simulink model "SF049A_LoaMgr"  (R2013b)
settings: Solver=FixedStepDiscrete  SolverMode=SingleTasking  StartTime=0.0  StopTime=1  FixedStep=0.002  RelTol=1e-3
undefined symbols (not defined in the file): CURRMEASLOAMTGTNMASK_CNT_U08, IVTRLOAMTGTNMASK_CNT_U08, LoaCtrldShtdwn, LoaCurrMeasIdptSigNrFlt, LoaHwTqIdptSigNrFlt, LoaImdtShtdwn, LoaIvtrIdptSigNrFlt, LOAMAXSLEW_ULSPERSEC_F32, LoaMgrCurrIvtrMtgtnRate, LoaMgrCurrIvtrMtgtnSca, LoaMgrCurrIvtrMtgtnScaZeroEna, LoaMgrCurrMeasIdptSig0Resp, LoaMgrCurrMeasIdptSig1Resp, LoaMgrCurrMeasIdptSig2Resp, LoaMgrCurrMeasIdptSigFltThd, LoaMgrCurrMeasMtgtnRate, LoaMgrCurrMeasMtgtnSca, LoaMgrCurrMeasMtgtnScaZeroEna, LoaMgrFadeOutStRate, LoaMgrHwTqIdptSig0NoTqLoaResp, LoaMgrHwTqIdptSig1NoTqLoaResp, LoaMgrHwTqIdptSig2Resp, LoaMgrHwTqIdptSig4Resp, LoaMgrHwTqIdptSigFltThd, LoaMgrHwTqLoaAvlResp, LoaMgrIvtrIdptSig0Resp, LoaMgrIvtrIdptSig1Resp, LoaMgrIvtrIdptSig2Resp, LoaMgrIvtrIdptSigFltThd, LoaMgrIvtrMtgtnRate, LoaMgrIvtrMtgtnSca, LoaMgrIvtrMtgtnScaZeroEna, LoaMgrLimdStRate, LoaMgrLimdStSca, LoaMgrMotAgAvlSnsrlsResp, LoaMgrMotAgIdptSig0NoSnsrlsResp, LoaMgrMotAgIdptSig1NoSnsrlsResp, LoaMgrMotAgIdptSig2Resp, LoaMgrMotAgIdptSig3Resp, LoaMgrMotAgIdptSigFltThd, LoaMgrMotAgMtgtnRate, LoaMgrMotAgMtgtnSca, LoaMgrMotAgMtgtnScaZeroEna, LoaMotAgIdptSigNrFlt, LOASCAONE_ULS_F32, LOASCAZERO_ULS_F32, LoaSt1, LOASTIMDTSHTDWN_CNT_U08, LOASTNORM_CNT_U08, LOASTSWMTGTN_CNT_U08, MAXCURRMEASIDPTSIGALLWD_CNT_U08, MAXHWTQIDPTSIGALLWD_CNT_U08, MAXIVTRIDPTSIGALLWD_CNT_U08, MAXMOTAGMECLIDPTSIGALLWD_CNT_U08, NODEBSTEP_CNT_U16, NtcSts1, SigQlfr1
libraries: simulink x30, NxtrMin x4, NxtrMax x4, NxtrLim x2
(part 5 of 7)

== system SF049A_LoaMgr/LoaMgr/LoaMgrPer1/Request_Responses/InvtrResp ==
  note: SWITCH IvtrIdptMin
      |     CASE 2
      |         CurrMeasResp = LoaMgrIvtrIdptSig2Resp
      |     CASE 1
      |          CurrMeasResp = LoaMgrIvtrIdptSig1Resp
      |     CASE ELSE
      |          CurrMeasResp = LoaMgrIvtrIdptSig0Resp
      | ENDSWITCH
  IvtrIdptMin : Inport  RequirementInfo={} %GIDa_2f7698e0_eca9_423b_adb0_11e1919669ef
  Constant : Constant  RequirementInfo="{'linktype_rmi_doors' '00012fd5 (/E-STEER Core/SubSystem Specifications/Application Functions - EA4/SF049A Loss of Assist Manager)' '#SF049A_128' 'true' 'REQ:  SF049A_128' '' } %GIDa_c2727e40_acbb_4c51_8514_00a2f788091d"  Value=LoaMgrIvtrIdptSig2Resp
  Constant1 : Constant  RequirementInfo="{'linktype_rmi_doors' '00012fd5 (/E-STEER Core/SubSystem Specifications/Application Functions - EA4/SF049A Loss of Assist Manager)' '#SF049A_128' 'true' 'REQ:  SF049A_128' '' } %GIDa_9020f9ee_b1a9_4c7e_bd34_28530cfb2ca8"  Value=LoaMgrIvtrIdptSig1Resp
  Constant2 : Constant  RequirementInfo="{'linktype_rmi_doors' '00012fd5 (/E-STEER Core/SubSystem Specifications/Application Functions - EA4/SF049A Loss of Assist Manager)' '#SF049A_128' 'true' 'REQ:  SF049A_128' '' } %GIDa_e0ea4ff4_d281_47bc_ab32_13335c3cc295"  Value=LoaMgrIvtrIdptSig0Resp
  CopyRight2 : Subsystem  Description=|  mask(Copyright Information){none=on}
      | Copyright info block.                                               
      |                                                                     
      | Place copyright information at the top of every subsystem in design.
      mask prompts: none "No parameters"
      mask help: Place copyright information at the top of every subsystem in design.
      mask Display:
      | NxtrConf = 'Nexteer Confidential';
      | 
      | sys = bdroot; %handle for the current model ("system")
      | first = get_param(sys,'Created');
      | first = first(end-3:end);  %year is last four digits
      | 
      | last = get_param(sys,'LastModifiedDate');
      | if isempty(last)
      |     last = datestr(now,'yyyy');
      | else
      |     last = last(end-3:end);
      | end
      | 
      | if strcmp(first,last)
      |     fprintf('%s -- Copyright %s Nexteer',NxtrConf,first)
      | else
      |     fprintf('%s -- %s%s- %s Nexteer',NxtrConf,char(169),first,last)
      | end
  Merge1 : Merge  RequirementInfo="{'linktype_rmi_doors' '00012fd5 (/E-STEER Core/SubSystem Specifications/Application Functions - EA4/SF049A Loss of Assist Manager)' '#SF049A_128' 'true' 'REQ:  SF049A_128' '' } %GIDa_78b8a886_be91_4ebf_bbb2_4a3f773a65b8"  Inputs=3
  Switch Case : SwitchCase  RequirementInfo="{'linktype_rmi_doors' '00012fd5 (/E-STEER Core/SubSystem Specifications/Application Functions - EA4/SF049A Loss of Assist Manager)' '#SF049A_128' 'true' 'REQ:  SF049A_128' '' } %GIDa_7dd0a01d_5238_4297_9e65_c2776d38f2c2"  CaseConditions={2,1}
  Two : Subsystem  RequirementInfo="{'linktype_rmi_doors' '00012fd5 (/E-STEER Core/SubSystem Specifications/Application Functions - EA4/SF049A Loss of Assist Manager)' '#SF049A_128' 'true' 'REQ:  SF049A_128' '' } %GIDa_c3edb1a4_418a_4dbd_ad2e_bc39f72c3322"  TreatAsAtomicUnit=on
      settings: RTWSystemCode=Inline
  Zero_or_Invalid : Subsystem  RequirementInfo="{'linktype_rmi_doors' '00012fd5 (/E-STEER Core/SubSystem Specifications/Application Functions - EA4/SF049A Loss of Assist Manager)' '#SF049A_128' 'true' 'REQ:  SF049A_128' '' } %GIDa_983bbd18_6fcb_4acf_ae46_7dfac766ba14"  TreatAsAtomicUnit=on
      settings: RTWSystemCode=Inline
  one : Subsystem  RequirementInfo="{'linktype_rmi_doors' '00012fd5 (/E-STEER Core/SubSystem Specifications/Application Functions - EA4/SF049A Loss of Assist Manager)' '#SF049A_128' 'true' 'REQ:  SF049A_128' '' } %GIDa_471ea5d0_5538_4611_a399_6254071c5581"  TreatAsAtomicUnit=on
      settings: RTWSystemCode=Inline
  IvtrResp : Outport  RequirementInfo={} %GIDa_f74e5785_bb35_4895_9ffd_742738152907
  wires:
  IvtrIdptMin/1 -> Switch Case/1
  Switch Case/3 -> Zero_or_Invalid/Action
  Switch Case/1 -> Two/Action
  Constant/1 -> Two/1(Sig2Resp)
  Switch Case/2 -> one/Action
  Constant1/1 -> one/1(Sig1Resp)
  Two/1(IvtrResp) -> Merge1/1
  one/1(IvtrResp) -> Merge1/2
  Merge1/1 -> IvtrResp/1
  Zero_or_Invalid/1(IvtrResp) -> Merge1/3
  Constant2/1 -> Zero_or_Invalid/1(Sig0Resp)

== system SF049A_LoaMgr/LoaMgr/LoaMgrPer1/Request_Responses/MotAgResp ==
  note: SWITCH MotPosnActvMin
      |     CASE 3
      |         MotAgResp = LoaMgrMotAgIdptSig3Resp
      |     CASE 2
      |         MotAgResp = LoaMgrMotAgIdptSig2Resp
      |     CASE 1
      |         IF SnsrlsMotAgAvl == true
      |             MotAgResp = LoaMgrMotAgAvlSnsrlsResp
      |         ELSE
      |             MotAgResp = LoaMgrMotAgIdptSig1NoSnsrlsResp
      |         ENDIF
      |     CASE ELSE
      |         IF SnsrlsMotAgAvl == true
      |             MotAgResp = LoaMgrMotAgAvlSnsrlsResp
      |         ELSE
      |             MotAgResp = LoaMgrMotAgIdptSig0NoSnsrlsResp
      |         ENDIF
      | ENDSWITCH
  MotAgIdptMin : Inport
  MotAgSnsrlsAvl : Inport  Port=2
  Constant : Constant  RequirementInfo="{'linktype_rmi_doors' '00012fd5 (/E-STEER Core/SubSystem Specifications/Application Functions - EA4/SF049A Loss of Assist Manager)' '#SF049A_123' 'true' 'REQ:  SF049A_123' '' } %GIDa_71dc042b_6702_4b9c_b0ca_6e7091752fa3"  Value=LoaMgrMotAgIdptSig3Resp
  Constant1 : Constant  RequirementInfo="{'linktype_rmi_doors' '00012fd5 (/E-STEER Core/SubSystem Specifications/Application Functions - EA4/SF049A Loss of Assist Manager)' '#SF049A_123' 'true' 'REQ:  SF049A_123' '' } %GIDa_c457ec65_eb6f_4051_8fe5_7ed6c1fa8831"  Value=LoaMgrMotAgIdptSig2Resp
  Constant2 : Constant  RequirementInfo="{'linktype_rmi_doors' '00012fd5 (/E-STEER Core/SubSystem Specifications/Application Functions - EA4/SF049A Loss of Assist Manager)' '#SF049A_123' 'true' 'REQ:  SF049A_123' '' } %GIDa_631a6b35_f334_47e8_b9e1_d44f002ffb93"  Value=LoaMgrMotAgAvlSnsrlsResp
  Constant3 : Constant  RequirementInfo="{'linktype_rmi_doors' '00012fd5 (/E-STEER Core/SubSystem Specifications/Application Functions - EA4/SF049A Loss of Assist Manager)' '#SF049A_123' 'true' 'REQ:  SF049A_123' '' } %GIDa_8db46fac_2835_4115_8682_627183a44b74"  Value=LoaMgrMotAgIdptSig1NoSnsrlsResp
  Constant4 : Constant  RequirementInfo="{'linktype_rmi_doors' '00012fd5 (/E-STEER Core/SubSystem Specifications/Application Functions - EA4/SF049A Loss of Assist Manager)' '#SF049A_123' 'true' 'REQ:  SF049A_123' '' } %GIDa_f54e32f6_6d5f_4cae_bb83_d22ec9538e2c"  Value=LoaMgrMotAgAvlSnsrlsResp
  Constant5 : Constant  RequirementInfo="{'linktype_rmi_doors' '00012fd5 (/E-STEER Core/SubSystem Specifications/Application Functions - EA4/SF049A Loss of Assist Manager)' '#SF049A_123' 'true' 'REQ:  SF049A_123' '' } %GIDa_dd061bd0_66be_43a3_9c2a_35a369cc1145"  Value=LoaMgrMotAgIdptSig0NoSnsrlsResp
  CopyRight2 : Subsystem  Description=|  mask(Copyright Information){none=on}
      | Copyright info block.                                               
      |                                                                     
      | Place copyright information at the top of every subsystem in design.
      mask prompts: none "No parameters"
      mask help: Place copyright information at the top of every subsystem in design.
      mask Display:
      | NxtrConf = 'Nexteer Confidential';
      | 
      | sys = bdroot; %handle for the current model ("system")
      | first = get_param(sys,'Created');
      | first = first(end-3:end);  %year is last four digits
      | 
      | last = get_param(sys,'LastModifiedDate');
      | if isempty(last)
      |     last = datestr(now,'yyyy');
      | else
      |     last = last(end-3:end);
      | end
      | 
      | if strcmp(first,last)
      |     fprintf('%s -- Copyright %s Nexteer',NxtrConf,first)
      | else
      |     fprintf('%s -- %s%s- %s Nexteer',NxtrConf,char(169),first,last)
      | end
  Merge1 : Merge  RequirementInfo="{'linktype_rmi_doors' '00012fd5 (/E-STEER Core/SubSystem Specifications/Application Functions - EA4/SF049A Loss of Assist Manager)' '#SF049A_123' 'true' 'REQ:  SF049A_123' '' } %GIDa_fdc09fa2_0a01_44bd_b8be_50e33525d629"  Inputs=4
  Switch Case : SwitchCase  RequirementInfo="{'linktype_rmi_doors' '00012fd5 (/E-STEER Core/SubSystem Specifications/Application Functions - EA4/SF049A Loss of Assist Manager)' '#SF049A_123' 'true' 'REQ:  SF049A_123' '' } %GIDa_59430f90_024e_4148_a99a_49e6c745560c"  CaseConditions={3,2,1}
  Three : Subsystem  RequirementInfo="{'linktype_rmi_doors' '00012fd5 (/E-STEER Core/SubSystem Specifications/Application Functions - EA4/SF049A Loss of Assist Manager)' '#SF049A_123' 'true' 'REQ:  SF049A_123' '' } %GIDa_3babd6cd_0d75_4a8e_8148_dab4727f0014"  TreatAsAtomicUnit=on
      settings: RTWSystemCode=Inline
  Two : Subsystem  RequirementInfo="{'linktype_rmi_doors' '00012fd5 (/E-STEER Core/SubSystem Specifications/Application Functions - EA4/SF049A Loss of Assist Manager)' '#SF049A_123' 'true' 'REQ:  SF049A_123' '' } %GIDa_50f45a0b_f423_489c_a78a_ec96fcd68be6"  TreatAsAtomicUnit=on
      settings: RTWSystemCode=Inline
  Zero_or_Invalid : Subsystem  RequirementInfo="{'linktype_rmi_doors' '00012fd5 (/E-STEER Core/SubSystem Specifications/Application Functions - EA4/SF049A Loss of Assist Manager)' '#SF049A_123' 'true' 'REQ:  SF049A_123' '' } %GIDa_417ac062_abea_453e_b11b_2ef37c8aa5f5"  TreatAsAtomicUnit=on
      settings: RTWSystemCode=Inline
  one : Subsystem  RequirementInfo="{'linktype_rmi_doors' '00012fd5 (/E-STEER Core/SubSystem Specifications/Application Functions - EA4/SF049A Loss of Assist Manager)' '#SF049A_123' 'true' 'REQ:  SF049A_123' '' } %GIDa_f7e2ee95_7d47_4ee5_b6c3_c744a2e7f7ac"  TreatAsAtomicUnit=on
      settings: RTWSystemCode=Inline
  MotAgResp : Outport  RequirementInfo={} %GIDa_506e1f0e_ad5f_4766_87b0_ff7db64cc3ed
  wires:
  Switch Case/3 -> one/Action
  MotAgIdptMin/1 -> Switch Case/1
  Switch Case/4 -> Zero_or_Invalid/Action
  Switch Case/1 -> Three/Action
  Constant/1 -> Three/1(cal)
  Switch Case/2 -> Two/Action
  Constant1/1 -> Two/1(cal)
  Constant2/1 -> one/1(MotAgAvlSnsrlsResp)
  Constant3/1 -> one/2(MotAgIdptSig1NoResp)
  MotAgSnsrlsAvl/1 -> [MotAgSnsrlsAvl]
  [MotAgSnsrlsAvl] -> one/3(MotAgSnsrlsAvl)
  Constant4/1 -> Zero_or_Invalid/1(MotAgAvlSnsrlsResp)
  Constant5/1 -> Zero_or_Invalid/2(MotAgIdptSig0NoResp)
  [MotAgSnsrlsAvl] -> Zero_or_Invalid/3(MotAgSnsrlsAvl)
  Three/1(MotAgResp) -> Merge1/1
  Two/1(MotAgResp) -> Merge1/2
  one/1(MotAgResp) -> Merge1/3
  Zero_or_Invalid/1(MotAgResp) -> Merge1/4
  Merge1/1 -> MotAgResp/1

== system SF049A_LoaMgr/LoaMgr/LoaMgrPer1/Set_Faults/CopyRight2 ==

== system SF049A_LoaMgr/LoaMgr/LoaMgrPer1/Set_Faults/NTC_Fault1 ==
  NtcNr : Inport
  NtcStInfo : Inport  Port=2
  NtcSts : Inport  Port=3
  DebStep : Inport  Port=4
  CallDiagMgr : ActionPort  ActionType=then
  SetNtcSts : Subsystem  RequirementInfo={} %GIDa_8b0d2f4e_7681_4688_a201_97bab6234a18  TreatAsAtomicUnit=on
      settings: RTWSystemCode=Inline
  wires:
  NtcStInfo/1 -> SetNtcSts/2(NtcStInfo)
  DebStep/1 -> SetNtcSts/4(DebStep)
  NtcSts/1 -> SetNtcSts/3(NtcSts)
  NtcNr/1 -> SetNtcSts/1(NtcNr)  "NtcNr"

== system SF049A_LoaMgr/LoaMgr/LoaMgrPer1/Set_Faults/NTC_Fault2 ==
  NtcNr : Inport
  NtcStInfo : Inport  Port=2
  NtcSts : Inport  Port=3
  DebStep : Inport  Port=4
  CallDiagMgr : ActionPort  ActionType=elseif
  SetNtcSts : Subsystem  RequirementInfo={} %GIDa_204fe94c_de92_4b33_aff5_e9c88726cf2c  TreatAsAtomicUnit=on
      settings: RTWSystemCode=Inline
  wires:
  NtcNr/1 -> SetNtcSts/1(NtcNr)  "NtcNr"
  NtcSts/1 -> SetNtcSts/3(NtcSts)
  DebStep/1 -> SetNtcSts/4(DebStep)
  NtcStInfo/1 -> SetNtcSts/2(NtcStInfo)

== system SF049A_LoaMgr/LoaMgr/LoaMgrPer1/Set_Faults/NTC_Fault3 ==
  NtcNr : Inport
  NtcStInfo : Inport  Port=2
  NtcSts : Inport  Port=3
  DebStep : Inport  Port=4
  CallDiagMgr : ActionPort  ActionType=then
  SetNtcSts : Subsystem  RequirementInfo={} %GIDa_37ef42c4_4520_4c9d_a45e_6bd4f10231da  TreatAsAtomicUnit=on
      settings: RTWSystemCode=Inline
  wires:
  NtcNr/1 -> SetNtcSts/1(NtcNr)  "NtcNr"
  NtcSts/1 -> SetNtcSts/3(NtcSts)
  DebStep/1 -> SetNtcSts/4(DebStep)
  NtcStInfo/1 -> SetNtcSts/2(NtcStInfo)

== system SF049A_LoaMgr/LoaMgr/LoaMgrPer1/Set_Faults/NTC_Fault4 ==
  NtcNr : Inport
  NtcStInfo : Inport  Port=2
  NtcSts : Inport  Port=3
  DebStep : Inport  Port=4
  CallDiagMgr : ActionPort  ActionType=then
  SetNtcSts : Subsystem  RequirementInfo={} %GIDa_b41b23fe_cdab_427f_85b1_ba14df8b4430  TreatAsAtomicUnit=on
      settings: RTWSystemCode=Inline
  wires:
  NtcStInfo/1 -> SetNtcSts/2(NtcStInfo)
  DebStep/1 -> SetNtcSts/4(DebStep)
  NtcSts/1 -> SetNtcSts/3(NtcSts)
  NtcNr/1 -> SetNtcSts/1(NtcNr)  "NtcNr"

== system SF049A_LoaMgr/LoaMgr/LoaMgrPer1/Set_Faults/NTC_Fault5 ==
  NtcNr : Inport
  NtcStInfo : Inport  Port=2
  NtcSts : Inport  Port=3
  DebStep : Inport  Port=4
  CallDiagMgr : ActionPort  ActionType=then
  CopyRight2 : Subsystem  Description=|  mask(Copyright Information){none=on}
      | Copyright info block.                                               
      |                                                                     
      | Place copyright information at the top of every subsystem in design.
      mask prompts: none "No parameters"
      mask help: Place copyright information at the top of every subsystem in design.
      mask Display:
      | NxtrConf = 'Nexteer Confidential';
      | 
      | sys = bdroot; %handle for the current model ("system")
      | first = get_param(sys,'Created');
      | first = first(end-3:end);  %year is last four digits
      | 
      | last = get_param(sys,'LastModifiedDate');
      | if isempty(last)
      |     last = datestr(now,'yyyy');
      | else
      |     last = last(end-3:end);
      | end
      | 
      | if strcmp(first,last)
      |     fprintf('%s -- Copyright %s Nexteer',NxtrConf,first)
      | else
      |     fprintf('%s -- %s%s- %s Nexteer',NxtrConf,char(169),first,last)
      | end
  Data Store Write1 : DataStoreWrite  DataStoreName=DebStep
  Data Store Write3 : DataStoreWrite  DataStoreName=Fault5_Status
  Terminator : Terminator
  Terminator1 : Terminator
  wires:
  NtcNr/1 -> Terminator/1
  NtcSts/1 -> Data Store Write3/1
  DebStep/1 -> Data Store Write1/1
  NtcStInfo/1 -> Terminator1/1

== system SF049A_LoaMgr/LoaMgr/LoaMgrPer1/Set_Faults/NTC_Fault6 ==
  NtcNr : Inport
  NtcStInfo : Inport  Port=2
  NtcSts : Inport  Port=3
  DebStep : Inport  Port=4
  CallDiagMgr : ActionPort  ActionType=then
  CopyRight2 : Subsystem  Description=|  mask(Copyright Information){none=on}
      | Copyright info block.                                               
      |                                                                     
      | Place copyright information at the top of every subsystem in design.
      mask prompts: none "No parameters"
      mask help: Place copyright information at the top of every subsystem in design.
      mask Display:
      | NxtrConf = 'Nexteer Confidential';
      | 
      | sys = bdroot; %handle for the current model ("system")
      | first = get_param(sys,'Created');
      | first = first(end-3:end);  %year is last four digits
      | 
      | last = get_param(sys,'LastModifiedDate');
      | if isempty(last)
      |     last = datestr(now,'yyyy');
      | else
      |     last = last(end-3:end);
      | end
      | 
      | if strcmp(first,last)
      |     fprintf('%s -- Copyright %s Nexteer',NxtrConf,first)
      | else
      |     fprintf('%s -- %s%s- %s Nexteer',NxtrConf,char(169),first,last)
      | end
  Data Store Write1 : DataStoreWrite  DataStoreName=DebStep
  Data Store Write3 : DataStoreWrite  DataStoreName=Fault6_Status
  Terminator : Terminator
  Terminator1 : Terminator
  wires:
  NtcStInfo/1 -> Terminator1/1
  DebStep/1 -> Data Store Write1/1
  NtcSts/1 -> Data Store Write3/1
  NtcNr/1 -> Terminator/1

== system SF049A_LoaMgr/ISO Fault Debounce/DiagMgr/NTCSTS_PREFAILD/If Action Subsystem1/CopyRight2 ==

== system SF049A_LoaMgr/ISO Fault Debounce/DiagMgr/NTCSTS_PREFAILD/If Action Subsystem1/If Action Subsystem ==
  EA : Inport
  Qlf : Inport  Port=2
  Action Port : ActionPort  ActionType=then
  EAo : Outport
  Qlfo : Outport  Port=2
  wires:
  EA/1 -> EAo/1
  Qlf/1 -> Qlfo/1

== system SF049A_LoaMgr/ISO Fault Debounce/DiagMgr/NTCSTS_PREFAILD/If Action Subsystem1/If Action Subsystem1 ==
  EA : Inport
  Qlf : Inport  Port=2
  Action Port : ActionPort  ActionType=else
  EAo : Outport
  Qlfo : Outport  Port=2
  wires:
  EA/1 -> EAo/1
  Qlf/1 -> Qlfo/1

== system SF049A_LoaMgr/LoaMgr/LoaMgrInit1/NTC_Fault1/SetNtcSts/CopyRight2 ==

== system SF049A_LoaMgr/LoaMgr/LoaMgrInit1/NTC_Fault2/SetNtcSts/CopyRight2 ==

== system SF049A_LoaMgr/LoaMgr/LoaMgrInit1/NTC_Fault3/SetNtcSts/CopyRight2 ==

== system SF049A_LoaMgr/LoaMgr/LoaMgrInit1/NTC_Fault4/SetNtcSts/CopyRight2 ==

== system SF049A_LoaMgr/LoaMgr/LoaMgrInit1/NTC_Fault5/SetNtcSts/CopyRight2 ==

== system SF049A_LoaMgr/LoaMgr/LoaMgrInit1/NTC_Fault6/SetNtcSts/CopyRight2 ==

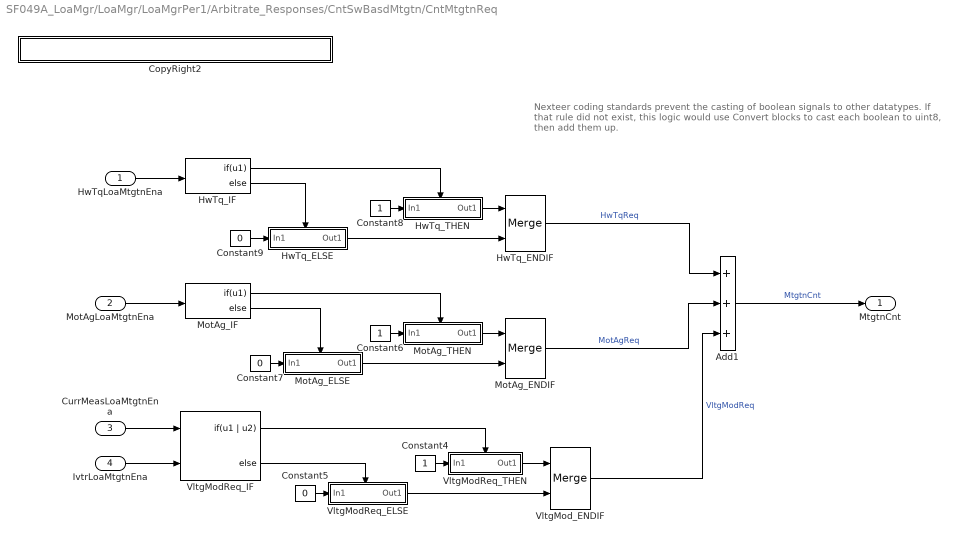
== system SF049A_LoaMgr/LoaMgr/LoaMgrPer1/Arbitrate_Responses/CntSwBasdMtgtn/CntMtgtnReq ==
  note: Nexteer coding standards prevent the casting of boolean signals to other datatypes.
      | If that rule did not exist, this logic would use Convert blocks to cast each boolean
      | to uint8, then add them up.
  HwTqLoaMtgtnEna : Inport  RequirementInfo={} %GIDa_468ac4b4_0a0c_481a_abf1_cf5448c64bfa
  MotAgLoaMtgtnEna : Inport  RequirementInfo={} %GIDa_2f6836a8_bec2_49a3_bf1d_79f90b25311f  Port=2
  CurrMeasLoaMtgtnEna : Inport  RequirementInfo={} %GIDa_5fb031fb_1f0b_4065_9016_e78b68d8bfa9  Port=3
  IvtrLoaMtgtnEna : Inport  RequirementInfo={} %GIDa_59799cc2_f2c7_40f5_82f7_91427f3a2199  Port=4
  Add1 : Sum  RequirementInfo="{'linktype_rmi_doors' '00012fd5 (/E-STEER Core/SubSystem Specifications/Application Functions - EA4/SF049A Loss of Assist Manager)' '#SF049A_166' 'true' 'REQ:  SF049A_166' '' } %GIDa_fc0e36f0_ea7b_4ef5_88c2_d0536a5d666e"  Inputs=+++
  Constant4 : Constant  RequirementInfo="{'linktype_rmi_doors' '00012fd5 (/E-STEER Core/SubSystem Specifications/Application Functions - EA4/SF049A Loss of Assist Manager)' '#SF049A_166' 'true' 'REQ:  SF049A_166' '' } %GIDa_3794e310_e42f_478d_81ca_b3774fc98e29"  OutDataTypeStr=uint8
      settings: AttributesFormatString=%<OutDataTypeStr>
  Constant5 : Constant  RequirementInfo="{'linktype_rmi_doors' '00012fd5 (/E-STEER Core/SubSystem Specifications/Application Functions - EA4/SF049A Loss of Assist Manager)' '#SF049A_166' 'true' 'REQ:  SF049A_166' '' } %GIDa_08550eda_19c6_4d71_8cfa_b34a1418c8b2"  Value=0  OutDataTypeStr=uint8
      settings: AttributesFormatString=%<OutDataTypeStr>
  Constant6 : Constant  RequirementInfo="{'linktype_rmi_doors' '00012fd5 (/E-STEER Core/SubSystem Specifications/Application Functions - EA4/SF049A Loss of Assist Manager)' '#SF049A_166' 'true' 'REQ:  SF049A_166' '' } %GIDa_c837754f_c7c3_40ec_8bc7_f06fc0e62241"  OutDataTypeStr=uint8
      settings: AttributesFormatString=%<OutDataTypeStr>
  Constant7 : Constant  RequirementInfo="{'linktype_rmi_doors' '00012fd5 (/E-STEER Core/SubSystem Specifications/Application Functions - EA4/SF049A Loss of Assist Manager)' '#SF049A_166' 'true' 'REQ:  SF049A_166' '' } %GIDa_2e085efc_cae7_441e_ae8f_e4cb8e5f5eaf"  Value=0  OutDataTypeStr=uint8
      settings: AttributesFormatString=%<OutDataTypeStr>
  Constant8 : Constant  RequirementInfo="{'linktype_rmi_doors' '00012fd5 (/E-STEER Core/SubSystem Specifications/Application Functions - EA4/SF049A Loss of Assist Manager)' '#SF049A_166' 'true' 'REQ:  SF049A_166' '' } %GIDa_32982a37_3a6c_4bcb_b890_9eab5f18d971"  OutDataTypeStr=uint8
      settings: AttributesFormatString=%<OutDataTypeStr>
  Constant9 : Constant  RequirementInfo="{'linktype_rmi_doors' '00012fd5 (/E-STEER Core/SubSystem Specifications/Application Functions - EA4/SF049A Loss of Assist Manager)' '#SF049A_166' 'true' 'REQ:  SF049A_166' '' } %GIDa_b6e29dd5_3368_40b8_87b0_603e90064365"  Value=0  OutDataTypeStr=uint8
      settings: AttributesFormatString=%<OutDataTypeStr>
  CopyRight2 : Subsystem  Description=|  mask(Copyright Information){none=on}
      | Copyright info block.                                               
      |                                                                     
      | Place copyright information at the top of every subsystem in design.
      mask prompts: none "No parameters"
      mask help: Place copyright information at the top of every subsystem in design.
      mask Display:
      | NxtrConf = 'Nexteer Confidential';
      | 
      | sys = bdroot; %handle for the current model ("system")
      | first = get_param(sys,'Created');
      | first = first(end-3:end);  %year is last four digits
      | 
      | last = get_param(sys,'LastModifiedDate');
      | if isempty(last)
      |     last = datestr(now,'yyyy');
      | else
      |     last = last(end-3:end);
      | end
      | 
      | if strcmp(first,last)
      |     fprintf('%s -- Copyright %s Nexteer',NxtrConf,first)
      | else
      |     fprintf('%s -- %s%s- %s Nexteer',NxtrConf,char(169),first,last)
      | end
  HwTq_ELSE : Subsystem  RequirementInfo="{'linktype_rmi_doors' '00012fd5 (/E-STEER Core/SubSystem Specifications/Application Functions - EA4/SF049A Loss of Assist Manager)' '#SF049A_166' 'true' 'REQ:  SF049A_166' '' } %GIDa_d76318f4_7c5f_4437_b67c_6e77cedc8b89"  TreatAsAtomicUnit=on
      settings: RTWSystemCode=Inline
  HwTq_ENDIF : Merge  RequirementInfo="{'linktype_rmi_doors' '00012fd5 (/E-STEER Core/SubSystem Specifications/Application Functions - EA4/SF049A Loss of Assist Manager)' '#SF049A_166' 'true' 'REQ:  SF049A_166' '' } %GIDa_571e4f8c_7894_44d6_89d8_dbaf55d6cadc"
  HwTq_IF : If  RequirementInfo="{'linktype_rmi_doors' '00012fd5 (/E-STEER Core/SubSystem Specifications/Application Functions - EA4/SF049A Loss of Assist Manager)' '#SF049A_166' 'true' 'REQ:  SF049A_166' '' } %GIDa_93ae7cfc_65c1_4d81_9733_91b95d8c5297"  IfExpression=u1
  HwTq_THEN : Subsystem  RequirementInfo="{'linktype_rmi_doors' '00012fd5 (/E-STEER Core/SubSystem Specifications/Application Functions - EA4/SF049A Loss of Assist Manager)' '#SF049A_166' 'true' 'REQ:  SF049A_166' '' } %GIDa_c3479270_c7a8_4f63_b2e0_e284767f7a06"  TreatAsAtomicUnit=on
      settings: RTWSystemCode=Inline
  MotAg_ELSE : Subsystem  RequirementInfo="{'linktype_rmi_doors' '00012fd5 (/E-STEER Core/SubSystem Specifications/Application Functions - EA4/SF049A Loss of Assist Manager)' '#SF049A_166' 'true' 'REQ:  SF049A_166' '' } %GIDa_55502f06_9f96_43ed_b305_2aaa83cf0cc1"  TreatAsAtomicUnit=on
      settings: RTWSystemCode=Inline
  MotAg_ENDIF : Merge  RequirementInfo="{'linktype_rmi_doors' '00012fd5 (/E-STEER Core/SubSystem Specifications/Application Functions - EA4/SF049A Loss of Assist Manager)' '#SF049A_166' 'true' 'REQ:  SF049A_166' '' } %GIDa_5cfeda37_4ca0_4c7d_91af_4d9483c27971"
  MotAg_IF : If  RequirementInfo="{'linktype_rmi_doors' '00012fd5 (/E-STEER Core/SubSystem Specifications/Application Functions - EA4/SF049A Loss of Assist Manager)' '#SF049A_166' 'true' 'REQ:  SF049A_166' '' } %GIDa_592f088d_e4ec_4e6b_98c3_76a1d7b711ea"  IfExpression=u1
  MotAg_THEN : Subsystem  RequirementInfo="{'linktype_rmi_doors' '00012fd5 (/E-STEER Core/SubSystem Specifications/Application Functions - EA4/SF049A Loss of Assist Manager)' '#SF049A_166' 'true' 'REQ:  SF049A_166' '' } %GIDa_e3b6c11b_0461_4c01_a62f_8b560565093f"  TreatAsAtomicUnit=on
      settings: RTWSystemCode=Inline
  VltgModReq_ELSE : Subsystem  RequirementInfo="{'linktype_rmi_doors' '00012fd5 (/E-STEER Core/SubSystem Specifications/Application Functions - EA4/SF049A Loss of Assist Manager)' '#SF049A_166' 'true' 'REQ:  SF049A_166' '' } %GIDa_2c14b666_cffc_4a3f_9f3c_8fd896b7e774"  TreatAsAtomicUnit=on
      settings: RTWSystemCode=Inline
  VltgModReq_IF : If  RequirementInfo="{'linktype_rmi_doors' '00012fd5 (/E-STEER Core/SubSystem Specifications/Application Functions - EA4/SF049A Loss of Assist Manager)' '#SF049A_166' 'true' 'REQ:  SF049A_166' '' } %GIDa_de65962a_d56f_4e30_aab1_150815f33c58"  NumInputs=2  IfExpression=u1 | u2
  VltgModReq_THEN : Subsystem  RequirementInfo="{'linktype_rmi_doors' '00012fd5 (/E-STEER Core/SubSystem Specifications/Application Functions - EA4/SF049A Loss of Assist Manager)' '#SF049A_166' 'true' 'REQ:  SF049A_166' '' } %GIDa_033ba68c_ccfd_49c6_b005_8c32e83e3980"  TreatAsAtomicUnit=on
      settings: RTWSystemCode=Inline
  VltgMod_ENDIF : Merge  RequirementInfo="{'linktype_rmi_doors' '00012fd5 (/E-STEER Core/SubSystem Specifications/Application Functions - EA4/SF049A Loss of Assist Manager)' '#SF049A_166' 'true' 'REQ:  SF049A_166' '' } %GIDa_11656fd0_98aa_47e4_b001_b40d4e0b90c9"
  MtgtnCnt : Outport  RequirementInfo={} %GIDa_287a12b5_618e_4d83_973e_837a98723898
  wires:
  VltgModReq_IF/2 -> VltgModReq_ELSE/Action
  VltgModReq_IF/1 -> VltgModReq_THEN/Action
  VltgMod_ENDIF/1 -> Add1/3  "VltgModReq"
  Add1/1 -> MtgtnCnt/1  "MtgtnCnt"
  HwTq_ENDIF/1 -> Add1/1  "HwTqReq"
  MotAg_ENDIF/1 -> Add1/2  "MotAgReq"
  CurrMeasLoaMtgtnEna/1 -> VltgModReq_IF/1
  IvtrLoaMtgtnEna/1 -> VltgModReq_IF/2
  Constant4/1 -> VltgModReq_THEN/1(In1)
  Constant5/1 -> VltgModReq_ELSE/1(In1)
  VltgModReq_THEN/1(Out1) -> VltgMod_ENDIF/1
  VltgModReq_ELSE/1(Out1) -> VltgMod_ENDIF/2
  MotAg_IF/2 -> MotAg_ELSE/Action
  MotAg_IF/1 -> MotAg_THEN/Action
  Constant6/1 -> MotAg_THEN/1(In1)
  Constant7/1 -> MotAg_ELSE/1(In1)
  MotAg_THEN/1(Out1) -> MotAg_ENDIF/1
  MotAg_ELSE/1(Out1) -> MotAg_ENDIF/2
  MotAgLoaMtgtnEna/1 -> MotAg_IF/1
  HwTq_IF/2 -> HwTq_ELSE/Action
  HwTq_IF/1 -> HwTq_THEN/Action
  Constant8/1 -> HwTq_THEN/1(In1)
  Constant9/1 -> HwTq_ELSE/1(In1)
  HwTq_THEN/1(Out1) -> HwTq_ENDIF/1
  HwTq_ELSE/1(Out1) -> HwTq_ENDIF/2
  HwTqLoaMtgtnEna/1 -> HwTq_IF/1

== system SF049A_LoaMgr/LoaMgr/LoaMgrPer1/Arbitrate_Responses/CntSwBasdMtgtn/CopyRight2 ==

== system SF049A_LoaMgr/LoaMgr/LoaMgrPer1/Arbitrate_Responses/CntSwBasdMtgtn/IllegalCombination ==
  note: Early drafts of this design used a calibration here.  Peer review team
      | preferred to hardcode an Immediate Shutdown until customer requirements
      | become more clear.
  Action Port : ActionPort  ActionType=else
  Constant2 : Constant  RequirementInfo={} %GIDa_ebd4b117_0579_4f87_9b11_dc243ea53af4  Value=LOASTIMDTSHTDWN_CNT_U08
  CopyRight2 : Subsystem  Description=|  mask(Copyright Information){none=on}
      | Copyright info block.                                               
      |                                                                     
      | Place copyright information at the top of every subsystem in design.
      mask prompts: none "No parameters"
      mask help: Place copyright information at the top of every subsystem in design.
      mask Display:
      | NxtrConf = 'Nexteer Confidential';
      | 
      | sys = bdroot; %handle for the current model ("system")
      | first = get_param(sys,'Created');
      | first = first(end-3:end);  %year is last four digits
      | 
      | last = get_param(sys,'LastModifiedDate');
      | if isempty(last)
      |     last = datestr(now,'yyyy');
      | else
      |     last = last(end-3:end);
      | end
      | 
      | if strcmp(first,last)
      |     fprintf('%s -- Copyright %s Nexteer',NxtrConf,first)
      | else
      |     fprintf('%s -- %s%s- %s Nexteer',NxtrConf,char(169),first,last)
      | end
  Out1 : Outport  RequirementInfo={} %GIDa_d7d4e985_f79e_4fcf_b3be_941c8d9ca7f4
  wires:
  Constant2/1 -> Out1/1

== system SF049A_LoaMgr/LoaMgr/LoaMgrPer1/Arbitrate_Responses/CntSwBasdMtgtn/OK_to_use ==
  Action Port : ActionPort  ActionType=then
  Constant : Constant  RequirementInfo={} %GIDa_4f56c85c_0d2e_4b56_bf9a_2b90391fffa9  Value=LOASTNORM_CNT_U08
  CopyRight2 : Subsystem  Description=|  mask(Copyright Information){none=on}
      | Copyright info block.                                               
      |                                                                     
      | Place copyright information at the top of every subsystem in design.
      mask prompts: none "No parameters"
      mask help: Place copyright information at the top of every subsystem in design.
      mask Display:
      | NxtrConf = 'Nexteer Confidential';
      | 
      | sys = bdroot; %handle for the current model ("system")
      | first = get_param(sys,'Created');
      | first = first(end-3:end);  %year is last four digits
      | 
      | last = get_param(sys,'LastModifiedDate');
      | if isempty(last)
      |     last = datestr(now,'yyyy');
      | else
      |     last = last(end-3:end);
      | end
      | 
      | if strcmp(first,last)
      |     fprintf('%s -- Copyright %s Nexteer',NxtrConf,first)
      | else
      |     fprintf('%s -- %s%s- %s Nexteer',NxtrConf,char(169),first,last)
      | end
  Out1 : Outport  RequirementInfo={} %GIDa_67551f9d_f493_4479_bacb_8cfa8f30743d
  wires:
  Constant/1 -> Out1/1

== system SF049A_LoaMgr/LoaMgr/LoaMgrPer1/Arbitrate_Responses/SelFinalResp/CopyRight2 ==

== system SF049A_LoaMgr/LoaMgr/LoaMgrPer1/Arbitrate_Responses/SelFinalResp/F1 ==
  F1 : ActionPort  ActionType=default
  CopyRight2 : Subsystem  Description=|  mask(Copyright Information){none=on}
      | Copyright info block.                                               
      |                                                                     
      | Place copyright information at the top of every subsystem in design.
      mask prompts: none "No parameters"
      mask help: Place copyright information at the top of every subsystem in design.
      mask Display:
      | NxtrConf = 'Nexteer Confidential';
      | 
      | sys = bdroot; %handle for the current model ("system")
      | first = get_param(sys,'Created');
      | first = first(end-3:end);  %year is last four digits
      | 
      | last = get_param(sys,'LastModifiedDate');
      | if isempty(last)
      |     last = datestr(now,'yyyy');
      | else
      |     last = last(end-3:end);
      | end
      | 
      | if strcmp(first,last)
      |     fprintf('%s -- Copyright %s Nexteer',NxtrConf,first)
      | else
      |     fprintf('%s -- %s%s- %s Nexteer',NxtrConf,char(169),first,last)
      | end
  Enumerated Constant : simulink/Sources/Enumerated Constant  OutDataTypeStr=Enum: LoaSt1  Value=LoaSt1.LOAST_IMDTSHTDWNREQD  SampleTime=inf
  LoaSt : Outport
  wires:
  Enumerated Constant/1 -> LoaSt/1

== system SF049A_LoaMgr/LoaMgr/LoaMgrPer1/Arbitrate_Responses/SelFinalResp/F2 ==
  F2 : ActionPort  ActionType=case
  CopyRight2 : Subsystem  Description=|  mask(Copyright Information){none=on}
      | Copyright info block.                                               
      |                                                                     
      | Place copyright information at the top of every subsystem in design.
      mask prompts: none "No parameters"
      mask help: Place copyright information at the top of every subsystem in design.
      mask Display:
      | NxtrConf = 'Nexteer Confidential';
      | 
      | sys = bdroot; %handle for the current model ("system")
      | first = get_param(sys,'Created');
      | first = first(end-3:end);  %year is last four digits
      | 
      | last = get_param(sys,'LastModifiedDate');
      | if isempty(last)
      |     last = datestr(now,'yyyy');
      | else
      |     last = last(end-3:end);
      | end
      | 
      | if strcmp(first,last)
      |     fprintf('%s -- Copyright %s Nexteer',NxtrConf,first)
      | else
      |     fprintf('%s -- %s%s- %s Nexteer',NxtrConf,char(169),first,last)
      | end
  Enumerated Constant : simulink/Sources/Enumerated Constant  OutDataTypeStr=Enum: LoaSt1  Value=LoaSt1.LOAST_CTRLDSHTDWNREQD  SampleTime=inf
  LoaSt : Outport
  wires:
  Enumerated Constant/1 -> LoaSt/1

== system SF049A_LoaMgr/LoaMgr/LoaMgrPer1/Arbitrate_Responses/SelFinalResp/Fade_Out ==
  F2 : ActionPort  ActionType=case
  CopyRight2 : Subsystem  Description=|  mask(Copyright Information){none=on}
      | Copyright info block.                                               
      |                                                                     
      | Place copyright information at the top of every subsystem in design.
      mask prompts: none "No parameters"
      mask help: Place copyright information at the top of every subsystem in design.
      mask Display:
      | NxtrConf = 'Nexteer Confidential';
      | 
      | sys = bdroot; %handle for the current model ("system")
      | first = get_param(sys,'Created');
      | first = first(end-3:end);  %year is last four digits
      | 
      | last = get_param(sys,'LastModifiedDate');
      | if isempty(last)
      |     last = datestr(now,'yyyy');
      | else
      |     last = last(end-3:end);
      | end
      | 
      | if strcmp(first,last)
      |     fprintf('%s -- Copyright %s Nexteer',NxtrConf,first)
      | else
      |     fprintf('%s -- %s%s- %s Nexteer',NxtrConf,char(169),first,last)
      | end
  Enumerated Constant : simulink/Sources/Enumerated Constant  OutDataTypeStr=Enum: LoaSt1  Value=LoaSt1.LOAST_FADEOUT  SampleTime=inf
  LoaSt : Outport
  wires:
  Enumerated Constant/1 -> LoaSt/1

== system SF049A_LoaMgr/LoaMgr/LoaMgrPer1/Arbitrate_Responses/SelFinalResp/Norm ==
  F2 : ActionPort  ActionType=case
  CopyRight2 : Subsystem  Description=|  mask(Copyright Information){none=on}
      | Copyright info block.                                               
      |                                                                     
      | Place copyright information at the top of every subsystem in design.
      mask prompts: none "No parameters"
      mask help: Place copyright information at the top of every subsystem in design.
      mask Display:
      | NxtrConf = 'Nexteer Confidential';
      | 
      | sys = bdroot; %handle for the current model ("system")
      | first = get_param(sys,'Created');
      | first = first(end-3:end);  %year is last four digits
      | 
      | last = get_param(sys,'LastModifiedDate');
      | if isempty(last)
      |     last = datestr(now,'yyyy');
      | else
      |     last = last(end-3:end);
      | end
      | 
      | if strcmp(first,last)
      |     fprintf('%s -- Copyright %s Nexteer',NxtrConf,first)
      | else
      |     fprintf('%s -- %s%s- %s Nexteer',NxtrConf,char(169),first,last)
      | end
  Enumerated Constant : simulink/Sources/Enumerated Constant  OutDataTypeStr=Enum: LoaSt1  Value=LoaSt1.LOAST_NORM  SampleTime=inf
  LoaSt : Outport
  wires:
  Enumerated Constant/1 -> LoaSt/1

== system SF049A_LoaMgr/LoaMgr/LoaMgrPer1/Arbitrate_Responses/SelFinalResp/Reduced ==
  F2 : ActionPort  ActionType=case
  CopyRight2 : Subsystem  Description=|  mask(Copyright Information){none=on}
      | Copyright info block.                                               
      |                                                                     
      | Place copyright information at the top of every subsystem in design.
      mask prompts: none "No parameters"
      mask help: Place copyright information at the top of every subsystem in design.
      mask Display:
      | NxtrConf = 'Nexteer Confidential';
      | 
      | sys = bdroot; %handle for the current model ("system")
      | first = get_param(sys,'Created');
      | first = first(end-3:end);  %year is last four digits
      | 
      | last = get_param(sys,'LastModifiedDate');
      | if isempty(last)
      |     last = datestr(now,'yyyy');
      | else
      |     last = last(end-3:end);
      | end
      | 
      | if strcmp(first,last)
      |     fprintf('%s -- Copyright %s Nexteer',NxtrConf,first)
      | else
      |     fprintf('%s -- %s%s- %s Nexteer',NxtrConf,char(169),first,last)
      | end
  Enumerated Constant : simulink/Sources/Enumerated Constant  OutDataTypeStr=Enum: LoaSt1  Value=LoaSt1.LOAST_LIMD  SampleTime=inf
  LoaSt : Outport
  wires:
  Enumerated Constant/1 -> LoaSt/1

== system SF049A_LoaMgr/LoaMgr/LoaMgrPer1/Arbitrate_Responses/SelFinalResp/SwBasd_Mtgtn ==
  F2 : ActionPort  ActionType=case
  CopyRight2 : Subsystem  Description=|  mask(Copyright Information){none=on}
      | Copyright info block.                                               
      |                                                                     
      | Place copyright information at the top of every subsystem in design.
      mask prompts: none "No parameters"
      mask help: Place copyright information at the top of every subsystem in design.
      mask Display:
      | NxtrConf = 'Nexteer Confidential';
      | 
      | sys = bdroot; %handle for the current model ("system")
      | first = get_param(sys,'Created');
      | first = first(end-3:end);  %year is last four digits
      | 
      | last = get_param(sys,'LastModifiedDate');
      | if isempty(last)
      |     last = datestr(now,'yyyy');
      | else
      |     last = last(end-3:end);
      | end
      | 
      | if strcmp(first,last)
      |     fprintf('%s -- Copyright %s Nexteer',NxtrConf,first)
      | else
      |     fprintf('%s -- %s%s- %s Nexteer',NxtrConf,char(169),first,last)
      | end
  Enumerated Constant : simulink/Sources/Enumerated Constant  OutDataTypeStr=Enum: LoaSt1  Value=LoaSt1.LOAST_SWBASDMTGTN  SampleTime=inf
  LoaSt : Outport
  wires:
  Enumerated Constant/1 -> LoaSt/1

== system SF049A_LoaMgr/LoaMgr/LoaMgrPer1/Assign_Scale/F1/CopyRight2 ==

== system SF049A_LoaMgr/LoaMgr/LoaMgrPer1/Assign_Scale/F2/CopyRight2 ==

== system SF049A_LoaMgr/LoaMgr/LoaMgrPer1/Assign_Scale/Fade/CopyRight2 ==

== system SF049A_LoaMgr/LoaMgr/LoaMgrPer1/Assign_Scale/Limd/CopyRight2 ==

== system SF049A_LoaMgr/LoaMgr/LoaMgrPer1/Assign_Scale/Norm/CopyRight2 ==

== system SF049A_LoaMgr/LoaMgr/LoaMgrPer1/Assign_Scale/SwMtgtn/CopyRight2 ==

== system SF049A_LoaMgr/LoaMgr/LoaMgrPer1/Assign_Scale/SwMtgtn/HwTqTrue ==
  Action Port : ActionPort  ActionType=then
  Constant1 : Constant  RequirementInfo={} %GIDa_e979227f_cfe6_4e3a_a5cf_430689d2d0d7  Value=LOAMAXSLEW_ULSPERSEC_F32
  Constant6 : Constant  RequirementInfo={} %GIDa_104183b9_405b_4e88_9173_b5e1effa84ac  Value=LOASCAONE_ULS_F32
  CopyRight2 : Subsystem  Description=|  mask(Copyright Information){none=on}
      | Copyright info block.                                               
      |                                                                     
      | Place copyright information at the top of every subsystem in design.
      mask prompts: none "No parameters"
      mask help: Place copyright information at the top of every subsystem in design.
      mask Display:
      | NxtrConf = 'Nexteer Confidential';
      | 
      | sys = bdroot; %handle for the current model ("system")
      | first = get_param(sys,'Created');
      | first = first(end-3:end);  %year is last four digits
      | 
      | last = get_param(sys,'LastModifiedDate');
      | if isempty(last)
      |     last = datestr(now,'yyyy');
      | else
      |     last = last(end-3:end);
      | end
      | 
      | if strcmp(first,last)
      |     fprintf('%s -- Copyright %s Nexteer',NxtrConf,first)
      | else
      |     fprintf('%s -- %s%s- %s Nexteer',NxtrConf,char(169),first,last)
      | end
  Sca : Outport  RequirementInfo={} %GIDa_e0a94cf6_b462_4b09_a0ec_0f98e07d4f58
  Rate : Outport  RequirementInfo={} %GIDa_def4c47a_4026_407b_a8e3_4f2182c475b7  Port=2
  wires:
  Constant1/1 -> Rate/1
  Constant6/1 -> Sca/1

== system SF049A_LoaMgr/LoaMgr/LoaMgrPer1/Assign_Scale/SwMtgtn/MaskBooleans ==
  note: value = 2
  note: value = 1
  note: Mask the booleans as integers with power of two values.  Add them to generate a temporary
      | variable whose value represents each unique combination of the two boolean inputs.
  CurrMeasLoaMtgtnEna : Inport  RequirementInfo={} %GIDa_a997a5b3_75eb_45c7_ae29_dfac2f9d4643
  IvtrLoaMtgtnEna : Inport  RequirementInfo={} %GIDa_88acce5f_06e8_41b3_8cf4_7ff19ae2b28e  Port=2
  Add1 : Sum  RequirementInfo={} %GIDa_38759ada_7c8d_4557_9779_cd619e630dfc
  Constant1 : Constant  RequirementInfo={} %GIDa_8fb24d71_a9a9_4106_9f3e_2744a1e1f162  Value=CURRMEASLOAMTGTNMASK_CNT_U08
  Constant2 : Constant  RequirementInfo={} %GIDa_6fa0fbbf_073c_42d4_a8db_2b337999c3ec  Value=0  OutDataTypeStr=uint8
  Constant5 : Constant  RequirementInfo={} %GIDa_d170084e_7ff2_445c_b3be_9b7206c269d6  Value=IVTRLOAMTGTNMASK_CNT_U08
  Constant6 : Constant  RequirementInfo={} %GIDa_e4f89cd4_562d_4984_9da1_365ee0a36b03  Value=0  OutDataTypeStr=uint8
  CopyRight2 : Subsystem  Description=|  mask(Copyright Information){none=on}
      | Copyright info block.                                               
      |                                                                     
      | Place copyright information at the top of every subsystem in design.
      mask prompts: none "No parameters"
      mask help: Place copyright information at the top of every subsystem in design.
      mask Display:
      | NxtrConf = 'Nexteer Confidential';
      | 
      | sys = bdroot; %handle for the current model ("system")
      | first = get_param(sys,'Created');
      | first = first(end-3:end);  %year is last four digits
      | 
      | last = get_param(sys,'LastModifiedDate');
      | if isempty(last)
      |     last = datestr(now,'yyyy');
      | else
      |     last = last(end-3:end);
      | end
      | 
      | if strcmp(first,last)
      |     fprintf('%s -- Copyright %s Nexteer',NxtrConf,first)
      | else
      |     fprintf('%s -- %s%s- %s Nexteer',NxtrConf,char(169),first,last)
      | end
  CurrMeas_ELSE : Subsystem  RequirementInfo={} %GIDa_b0d394bd_5bdb_4869_bfc4_608112a94472  TreatAsAtomicUnit=on
      settings: RTWSystemCode=Inline
  CurrMeas_IF : If  RequirementInfo={} %GIDa_6ae73889_b7ce_483e_91da_d116fc63b2d0  IfExpression=u1
  CurrMeas_THEN : Subsystem  RequirementInfo={} %GIDa_253bd3cf_a501_475f_9ccb_2e38fcd20341  TreatAsAtomicUnit=on
      settings: RTWSystemCode=Inline
  Ivtr_ELSE : Subsystem  RequirementInfo={} %GIDa_3bf7609c_b8a7_4203_bd13_c77d2e5548c4  TreatAsAtomicUnit=on
      settings: RTWSystemCode=Inline
  Ivtr_IF : If  RequirementInfo={} %GIDa_14670552_10c0_463d_a30f_3d5e71a6c41d  IfExpression=u1
  Ivtr_THEN : Subsystem  RequirementInfo={} %GIDa_aa80acd7_5c89_4d23_a000_4adaacefc61e  TreatAsAtomicUnit=on
      settings: RTWSystemCode=Inline
  Merge2 : Merge  RequirementInfo={} %GIDa_784b84a1_e1cc_4391_82ff_f6bd0e24e4bd
  Merge3 : Merge  RequirementInfo={} %GIDa_ac094152_cb86_4cd3_b3fb_fbe9a20e63e8
  VltgModSrc : Outport  RequirementInfo={} %GIDa_06805c96_75af_4704_9ff8_7153cb9b206f
  wires:
  IvtrLoaMtgtnEna/1 -> Ivtr_IF/1
  CurrMeasLoaMtgtnEna/1 -> CurrMeas_IF/1
  Add1/1 -> VltgModSrc/1
  Merge2/1 -> Add1/1
  CurrMeas_IF/2 -> CurrMeas_ELSE/Action
  Constant2/1 -> CurrMeas_ELSE/1(In1)
  Ivtr_IF/1 -> Ivtr_THEN/Action
  Ivtr_IF/2 -> Ivtr_ELSE/Action
  Constant5/1 -> Ivtr_THEN/1(In1)
  Constant6/1 -> Ivtr_ELSE/1(In1)
  Ivtr_ELSE/1(Out1) -> Merge3/2
  Ivtr_THEN/1(Out1) -> Merge3/1
  CurrMeas_THEN/1(Out1) -> Merge2/1
  Constant1/1 -> CurrMeas_THEN/1(In1)
  Merge3/1 -> Add1/2
  CurrMeas_ELSE/1(Out1) -> Merge2/2
  CurrMeas_IF/1 -> CurrMeas_THEN/Action

== system SF049A_LoaMgr/LoaMgr/LoaMgrPer1/Assign_Scale/SwMtgtn/MotAgTrue ==
  note: If we enter this block on the next loop, the state variable ("previous value") will already be
      | TRUE because of the current loop.  The user's calibrated scale factor and slew rate will
      | be used.  This means that the slew rate is applied whether the system is slewing down from
      | ONE or up from ZERO.
  note: We could only reach this routine when the new value is true
      | So if old value is false, it is our first time entering this block.
      | If the user wants to momentarily drop scale factor instantly to
      | zero, this transition from false to true is the time to do it.
  note: IF cal is true and previous value is false THEN
      |      Target scale factor is Zero
      |      Slew rate is instantaneous
      | ELSE
      |      Target scale factor is a cal value
      |      Slew rate is a cal value
      | ENDIF
  PrevMotAgLoaMtgtnEn : Inport  RequirementInfo={} %GIDa_5d35e019_f0d1_4617_8c1c_64a692c8181d
  Action Port : ActionPort  ActionType=elseif
  Constant1 : Constant  RequirementInfo={} %GIDa_1bdc5e56_3e02_4165_b6e0_38f2aaaea0cc  Value=LoaMgrMotAgMtgtnRate
  Constant2 : Constant  RequirementInfo={} %GIDa_01cc2f33_91ba_4788_b8fe_96c45da0786d  Value=LOASCAZERO_ULS_F32
  Constant3 : Constant  RequirementInfo={} %GIDa_61d17128_67a2_449a_aa6d_d426bb2e61a4  Value=LOAMAXSLEW_ULSPERSEC_F32
  Constant4 : Constant  RequirementInfo={} %GIDa_0e3d0a1c_66bf_432b_885d_72a46e89491d  Value=LoaMgrMotAgMtgtnScaZeroEna
  Constant6 : Constant  RequirementInfo={} %GIDa_847ef365_26bc_443f_a652_b6afa8fe4243  Value=LoaMgrMotAgMtgtnSca
  CopyRight2 : Subsystem  Description=|  mask(Copyright Information){none=on}
      | Copyright info block.                                               
      |                                                                     
      | Place copyright information at the top of every subsystem in design.
      mask prompts: none "No parameters"
      mask help: Place copyright information at the top of every subsystem in design.
      mask Display:
      | NxtrConf = 'Nexteer Confidential';
      | 
      | sys = bdroot; %handle for the current model ("system")
      | first = get_param(sys,'Created');
      | first = first(end-3:end);  %year is last four digits
      | 
      | last = get_param(sys,'LastModifiedDate');
      | if isempty(last)
      |     last = datestr(now,'yyyy');
      | else
      |     last = last(end-3:end);
      | end
      | 
      | if strcmp(first,last)
      |     fprintf('%s -- Copyright %s Nexteer',NxtrConf,first)
      | else
      |     fprintf('%s -- %s%s- %s Nexteer',NxtrConf,char(169),first,last)
      | end
  If : If  RequirementInfo={} %GIDa_a602bf6c_b97c_48d9_a82c_25a7d3776676  NumInputs=2  IfExpression=u2 & ~u1
  PassThru1 : Subsystem  RequirementInfo={} %GIDa_0d02e917_8845_4f36_9b2b_7c2f608afbcb  TreatAsAtomicUnit=on
      settings: RTWSystemCode=Inline
  PassThru2 : Subsystem  RequirementInfo={} %GIDa_b60de95f_d360_448a_abc2_c2c3a0e2400b  TreatAsAtomicUnit=on
      settings: RTWSystemCode=Inline
  RateMerge : Merge  RequirementInfo={} %GIDa_ab71ab8e_ab39_405c_99f2_6334510a7570
  ScaMerge : Merge  RequirementInfo={} %GIDa_87dfc468_6e08_4627_9309_01e2732dfdb5
  Sca : Outport  RequirementInfo={} %GIDa_a3e0ede8_75b2_4643_9c83_cdff2b1f8999
  Rate : Outport  RequirementInfo={} %GIDa_be2b081d_f81b_4fad_8c1b_b4cb94b7c82b  Port=2
  wires:
  PassThru2/2(Rate) -> RateMerge/2
  PassThru2/1(Sca) -> ScaMerge/2
  PassThru1/2(Rate) -> RateMerge/1
  PassThru1/1(Sca) -> ScaMerge/1
  If/2 -> PassThru2/Action
  If/1 -> PassThru1/Action
  Constant1/1 -> PassThru2/2(In2)
  Constant6/1 -> PassThru2/1(In1)
  Constant3/1 -> PassThru1/2(In2)
  Constant2/1 -> PassThru1/1(In1)
  Constant4/1 -> If/2
  PrevMotAgLoaMtgtnEn/1 -> If/1
  RateMerge/1 -> Rate/1
  ScaMerge/1 -> Sca/1
